simulink model "Cruise_Control"  (R2020a)
settings: Solver=ode45  StartTime=0.0  StopTime=120  RelTol=1e-3
PreLoadFcn:
  | Kp=22;
  | Ki=4.5;
  | Kd=3.6;
  | m = 1000 ;
  | b = 50 ;
  | u = 500;
settings Model: Creator=Ganesh  LastModifiedBy=Ganesh
settings DataIOCC: SaveOutput=off  SaveTime=off

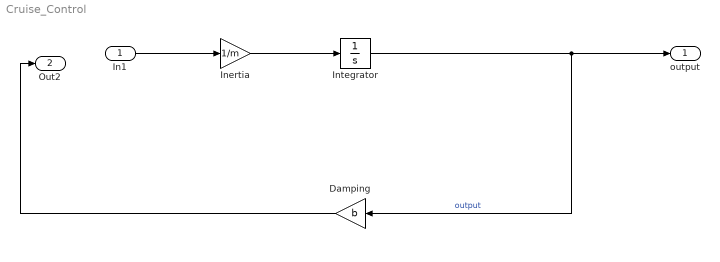
== system Cruise_Control ==
  In1 : Inport  OutDataTypeStr=double  PortDimensions=1  SampleTime=0
  Damping : Gain  Gain=b
  Inertia : Gain  Gain=1/m
  Integrator : Integrator
  output : Outport  OutDataTypeStr=double  PortDimensions=1  SampleTime=0
  Out2 : Outport  Port=2  OutDataTypeStr=double  PortDimensions=1  SampleTime=0
  wires:
  In1/1 -> Inertia/1
  Integrator/1 -> Damping/1, output/1  "output"
  Damping/1 -> Out2/1
  Inertia/1 -> Integrator/1
